simulink model "Uklad_Obiekt_Regulator_Obserwator"  (R2024a)
settings: Solver=VariableStepAuto  StartTime=0.0  StopTime=3  RelTol=1e-3
values from neighbouring files (symbols this model uses):
  K = K_r(1:end-1)    [oblicz_parametry_obserwatora_z_calkowaniem.m]    (also in oblicz_parametry_regulatora.m = acker(A, B, [s_b s_b s_b]); symulacjeObserwator.m = oblicz_parametry_regulatora(A, B, s_b); symulacjeObserwatorZero.m = oblicz_parametry_regulatora(A, B, s_b); symulacjeRegulator.m = oblicz_parametry_regulatora(A, B, s_b))
  L = acker(A', C', [s_o s_o s_o])'    [oblicz_parametry_obserwatora.m]    (also in symulacjeObserwator.m = oblicz_parametry_obserwatora(A, C, s_o); symulacjeObserwatorZero.m = oblicz_parametry_obserwatora(A, C, s_o); symulacjeRegulatorObserwator.m = oblicz_parametry_obserwatora(A, C, s_o))
  X_0 = [1; -5; 1]    [symulacjeObserwator.m]    (also in symulacjeObserwatorZero.m; symulacjeRegulator.m; symulacjeRegulatorCalka.m = [0; 0; 0]; symulacjeRegulatorCalka150.m = [0; 0; 0])
  Xd_0 = [10; 20; 30]    [symulacjeObserwator.m]    (also in symulacjeObserwatorZero.m = [0; 0; 0]; symulacjeRegulatorObserwator.m)
settings Model: Creator=pioro  LastModifiedBy=pioro
settings OptimizationCC: ReuseModelBlockBuffer=off
settings RTWCC: GPUComputeCapability=3.5

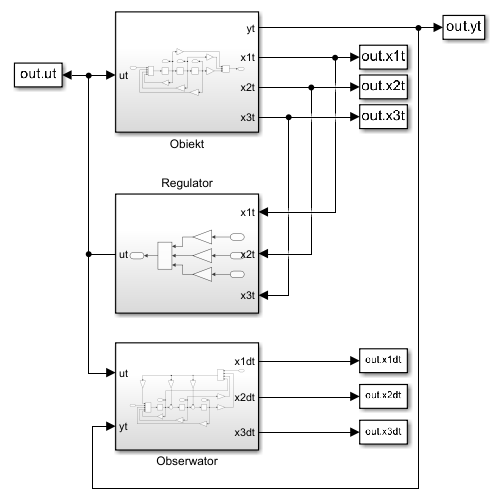
[thumbnail: Simulink's stored preview of the top-level diagram]
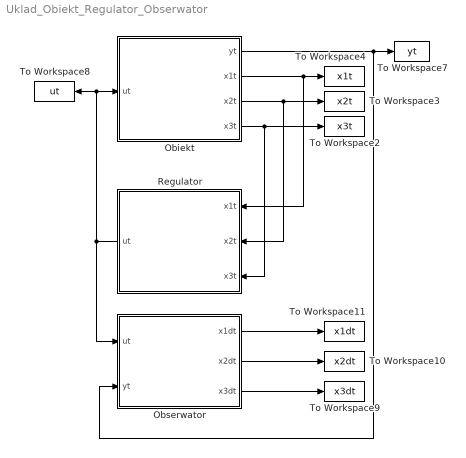
== system Uklad_Obiekt_Regulator_Obserwator ==
  Obiekt : Subsystem
  Obserwator : Subsystem
  Regulator : Subsystem
  To Workspace10 : ToWorkspace  VariableName=x2dt  SaveFormat=Timeseries  SampleTime=-1
  To Workspace11 : ToWorkspace  VariableName=x1dt  SaveFormat=Timeseries  SampleTime=-1
  To Workspace2 : ToWorkspace  VariableName=x3t  SaveFormat=Timeseries  SampleTime=-1
  To Workspace3 : ToWorkspace  VariableName=x2t  SaveFormat=Timeseries  SampleTime=-1
  To Workspace4 : ToWorkspace  VariableName=x1t  SaveFormat=Timeseries  SampleTime=-1
  To Workspace7 : ToWorkspace  VariableName=yt  SaveFormat=Timeseries  SampleTime=-1
  To Workspace8 : ToWorkspace  VariableName=ut  SaveFormat=Timeseries  SampleTime=-1
  To Workspace9 : ToWorkspace  VariableName=x3dt  SaveFormat=Timeseries  SampleTime=-1
  wires:
  Obiekt/3(x2t) -> To Workspace3/1, Regulator/2(x2t)
  Obiekt/2(x1t) -> To Workspace4/1, Regulator/1(x1t)
  Obiekt/4(x3t) -> To Workspace2/1, Regulator/3(x3t)
  Regulator/1(ut) -> Obserwator/1(ut), To Workspace8/1, Obiekt/1(ut)
  Obiekt/1(yt) -> To Workspace7/1, Obserwator/2(yt)
  Obserwator/1(x1dt) -> To Workspace11/1
  Obserwator/2(x2dt) -> To Workspace10/1
  Obserwator/3(x3dt) -> To Workspace9/1

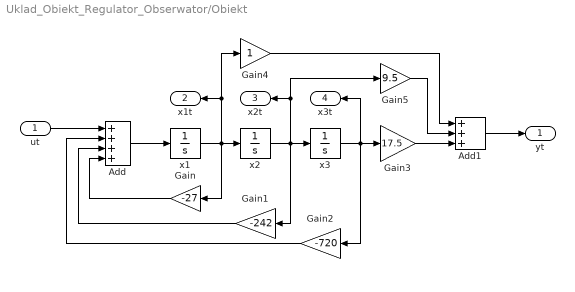
== system Uklad_Obiekt_Regulator_Obserwator/Obiekt ==
  ut : Inport
  Add : Sum  Inputs=++++
  Add1 : Sum  Inputs=+++
  Gain : Gain  Gain=-27
  Gain1 : Gain  Gain=-242
  Gain2 : Gain  Gain=-720
  Gain3 : Gain  Gain=17.5
  Gain4 : Gain
  Gain5 : Gain  Gain=9.5
  x1 : Integrator  InitialCondition=X_0(1)
  x2 : Integrator  InitialCondition=X_0(2)
  x3 : Integrator  InitialCondition=X_0(3)
  yt : Outport
  x1t : Outport  Port=2
  x2t : Outport  Port=3
  x3t : Outport  Port=4
  wires:
  x3/1 -> Gain2/1, Gain3/1, x3t/1
  ut/1 -> Add/1
  Gain4/1 -> Add1/1
  x1/1 -> Gain4/1, x1t/1, x2/1, Gain/1
  Gain1/1 -> Add/3
  Gain3/1 -> Add1/3
  Gain5/1 -> Add1/2
  Add1/1 -> yt/1
  Add/1 -> x1/1
  Gain2/1 -> Add/2
  Gain/1 -> Add/4
  x2/1 -> Gain5/1, x2t/1, x3/1, Gain1/1

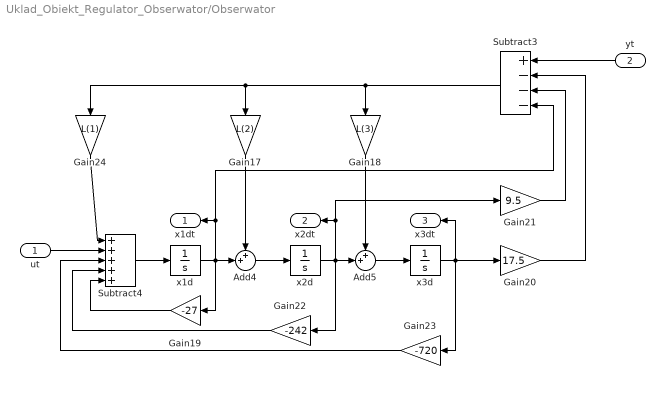
== system Uklad_Obiekt_Regulator_Obserwator/Obserwator ==
  ut : Inport
  yt : Inport  Port=2
  Add4 : Sum  Inputs=++|
  Add5 : Sum  Inputs=++|
  Gain17 : Gain  Gain=L(2)
  Gain18 : Gain  Gain=L(3)
  Gain19 : Gain  Gain=-27
  Gain20 : Gain  Gain=17.5
  Gain21 : Gain  Gain=9.5
  Gain22 : Gain  Gain=-242
  Gain23 : Gain  Gain=-720
  Gain24 : Gain  Gain=L(1)
  Subtract3 : Sum  Inputs=+---
  Subtract4 : Sum  Inputs=+++++
  x1d : Integrator  InitialCondition=Xd_0(1)
  x2d : Integrator  InitialCondition=Xd_0(2)
  x3d : Integrator  InitialCondition=Xd_0(3)
  x1dt : Outport
  x2dt : Outport  Port=2
  x3dt : Outport  Port=3
  wires:
  Gain19/1 -> Subtract4/5
  x3d/1 -> Gain23/1, Gain20/1, x3dt/1
  Subtract3/1 -> Gain24/1, Gain17/1, Gain18/1
  Gain17/1 -> Add4/1
  Gain20/1 -> Subtract3/2
  Gain21/1 -> Subtract3/3
  x2d/1 -> Add5/2, Gain22/1, x2dt/1, Gain21/1
  yt/1 -> Subtract3/1
  Gain23/1 -> Subtract4/3
  Gain18/1 -> Add5/1
  Add4/1 -> x2d/1
  x1d/1 -> Add4/2, Gain19/1, x1dt/1, Subtract3/4
  Subtract4/1 -> x1d/1
  Add5/1 -> x3d/1
  Gain22/1 -> Subtract4/4
  Gain24/1 -> Subtract4/1
  ut/1 -> Subtract4/2

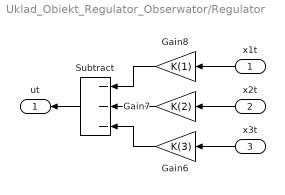
== system Uklad_Obiekt_Regulator_Obserwator/Regulator ==
  x1t : Inport
  x2t : Inport  Port=2
  x3t : Inport  Port=3
  Gain6 : Gain  Gain=K(3)
  Gain7 : Gain  Gain=K(2)
  Gain8 : Gain  Gain=K(1)
  Subtract : Sum  Inputs=---
  ut : Outport
  wires:
  Gain7/1 -> Subtract/2
  Gain6/1 -> Subtract/3
  Gain8/1 -> Subtract/1
  x3t/1 -> Gain6/1
  Subtract/1 -> ut/1
  x1t/1 -> Gain8/1
  x2t/1 -> Gain7/1
